simulink model "multiRobotExampleModel"  (R2019b)
settings: Solver=FixedStepAuto  StartTime=0.0  StopTime=inf  FixedStep=0.1  RelTol=1e-3
PreLoadFcn:
  | exampleMultiRobotHelperInit
InitFcn:
  | set_param('multiRobotExampleModel', 'ForceConsistencyChecking', 'off');
undefined symbols (not defined in the file): chargingStations, loadingStation, logicalMap, numRobots, packages, RobotState, unloadingStations
libraries: robotmobilelib x5
settings Model: Creator=The MathWorks, Inc.  LastModifiedBy=Helsi

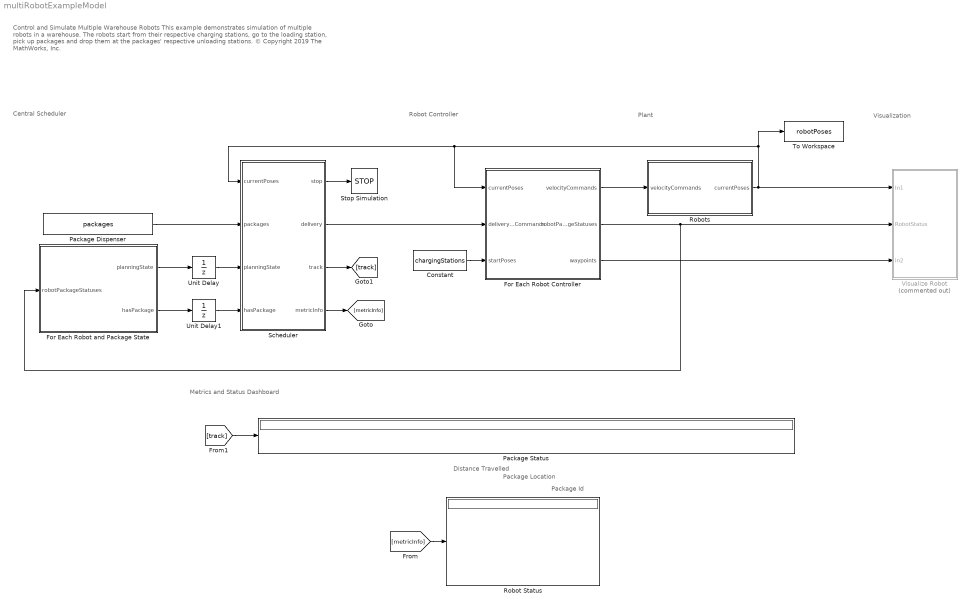
== system multiRobotExampleModel ==
  note: Visualization
  note: Plant
  note: Robot Controller
  note: Central Scheduler
  note: Metrics and Status Dashboard
  note: Package
      | Location
  note: Package Id
  note: Distance
      | Travelled
  note: Control and Simulate Multiple Warehouse Robots
      | This example demonstrates simulation of multiple robots in a warehouse. The robots start from their respective charging stations, go to the loading station, pick up packages and drop them at the packages' respective unloading stations.
      |
      | © Copyright 2019 The MathWorks, Inc.
  Constant : Constant  Value=chargingStations
  For Each Robot Controller : Subsystem  TreatAsAtomicUnit=on
  For Each Robot and Package State : Subsystem  TreatAsAtomicUnit=on
  Package Dispenser : Constant  Value=packages
  "Package Status " : Display
  Robot Status : Display
  Robots : Subsystem
  Scheduler : Stateflow chart  Priority=1  BlockKeywords=__PRM__SERIALIZED__DATA__:Stateflow Chart,Stateflow Diagram  TreatAsAtomicUnit=on
  Stop Simulation : Stop
  To Workspace : ToWorkspace  VariableName=robotPoses  SampleTime=-1
  Unit Delay : UnitDelay  InitialCondition=repmat(RobotState.AtDock, [1, numRobots])  SampleTime=-1  HasFrameUpgradeWarning=on
  Unit Delay1 : UnitDelay  InitialCondition=repmat(0, [1, numRobots])  SampleTime=-1  HasFrameUpgradeWarning=on
  Visualize Robot : Subsystem  Commented=on  mask{MeshSelectionIdx=Ground vehicle, PresetViews=Entire Map, ShowViz=on, ShowPaths=on, MapXMin=0, MapXMax=[], MapYMin=0, MapYMax=[], XLimits=[0 60], YLimits=[0 60], LocalXLimits=[-10 10], LocalYLimits=[-10 10], StartLocations=chargingStations, DockLocations=loadingStation, ShelfLocations=unloadingStations, VisualizationSampleRate=10}
      mask prompts: MeshSelectionIdx "Robot mesh"; PresetViews "Preset Views"; ShowViz "Update visualization:"; ShowPaths "Show planned paths:"; MapXMin "Map xmin:"; MapXMax "Map xmax:"; MapYMin "Map ymin:"; MapYMax "Map ymax:"; XLimits "Map x-limits:"; YLimits "Map y-limits:"; LocalXLimits "Local view x-limits"; LocalYLimits "Local view y-limits"; StartLocations "Start locations:"; DockLocations "Dock locations:"; ShelfLocations "Shelf locations:"; VisualizationSampleRate "Sample time:"
      mask init:
      | % Create the list of key locations
      | startLocationMatrix = evalin('base', get_param(gcb, 'StartLocations'));
      | shelfLocationMatrix = evalin('base', get_param(gcb, 'ShelfLocations'));
      | dockLocationMatrix = evalin('base', get_param(gcb, 'DockLocations'));
      | 
      | % Create popup list from matrices
      | dockLocationNameCell = cell(size(dockLocationMatrix,1),1);
      | shelfLocationNameCell = cell(size(shelfLocationMatrix,1),1);
      | startLocationNameCell = cell(size(startLocationMatrix,1),1);
      | for i = 1:size(startLocationMatrix,1)
      |     startLocationNameCell{i} = ['Start Location ' num2str(i)];
      | end
      | for j = 1:size(shelfLocationMatrix,1)
      |     shelfLocationNameCell{j} = ['Shelf Location ' num2str(j)];
      | end
      | for k = 1:size(dockLocationMatrix,1)
      |     dockLocationNameCell{k} = ['Dock Location ' num2str(k)];
      | end
      | 
      | % Update the parameter list
      | m = Simulink.Mask.get(gcb);
      | viewPopupParam = m.getParameter('PresetViews');
      | viewPopupParam.TypeOptions = [...
      |     {'Entire Map'}; ...
      |     dockLocationNameCell; ...
      |     shelfLocationNameCell; ...
      |     startLocationNameCell ... 
      |     ];
      mask TypeOptions MeshSelectionIdx: Ground vehicle | Forklift
      mask TypeOptions PresetViews: Entire Map | Dock Location 1 | Shelf Location 1 | Shelf Location 2 | Shelf Location 3 | Start Location 1 | Start Location 2 | Start Location 3 | Start Location 4 | Start Location 5
      mask Callback PresetViews:
      | % Get key numeric data
      | startLocationMatrix = evalin('base', get_param(gcb, 'StartLocations'));
      | dockLocationMatrix = evalin('base', get_param(gcb, 'DockLocations'));
      | shelfLocationMatrix = evalin('base', get_param(gcb, 'ShelfLocations'));
      | mapXLim = evalin('base', get_param(gcb, 'XLimits'));
      | mapYLim = evalin('base', get_param(gcb, 'YLimits'));
      | viewXLim = evalin('base', get_param(gcb, 'LocalXLimits'));
      | viewYLim = evalin('base', get_param(gcb, 'LocalYLimits'));
      | 
      | % Get selected value
      | viewSelection = get_param(gcb, 'PresetViews');
      | 
      | % Take action based on view
      | if strcmp(viewSelection, 'Custom')
      |     % Do nothing
      | else
      |     if strcmp(viewSelection(1:5), 'Start')
      |         % Start location
      |         startIndex = str2double(viewSelection(16:end));
      |         localPts = startLocationMatrix(startIndex, :);
      |         viewLimits = [localPts(1)+viewXLim(1) localPts(1)+viewXLim(2) ...
      |             localPts(2)+viewYLim(1) localPts(2)+viewYLim(2)];
      | 
      |     elseif strcmp(viewSelection(1:5), 'Dock ')
      |         % Dock (Loading) location
      |         dockIndex = str2double(viewSelection(15:end));
      |         localPts = dockLocationMatrix(dockIndex, :);
      |         viewLimits = [localPts(1)+viewXLim(1) localPts(1)+viewXLim(2) ...
      |             localPts(2)+viewYLim(1) localPts(2)+viewYLim(2)];
      | 
      |     elseif strcmp(viewSelection(1:5), 'Shelf')
      |         % Shelf (Unloading) location
      |         shelfIndex = str2double(viewSelection(16:end));
      |         localPts = shelfLocationMatrix(shelfIndex, :);
      |         viewLimits = [localPts(1)+viewXLim(1) localPts(1)+viewXLim(2) ...
      |             localPts(2)+viewYLim(1) localPts(2)+viewYLim(2)];
      | 
      |     else
      |         % Show the whole map
      |         viewLimits = [mapXLim(1) mapXLim(2) mapYLim(1) mapYLim(2)];
      |     end
      | 
      |     % Set the map parameters
      |     set_param(gcb, 'MapXMin', num2str(viewLimits(1)));
      |     set_param(gcb, 'MapXMax', num2str(viewLimits(2)));
      |     set_param(gcb, 'MapYMin', num2str(viewLimits(3)));
      |     set_param(gcb, 'MapYMax', num2str(viewLimits(4)));
      | end
      mask Callback MapXMin:
      | currentMax = str2num(get_param(gcb, 'MapXMax'));
      | newMin = str2num(get_param(gcb, 'MapXMin'));
      | if newMin > currentMax
      |     set_param(gcb, 'MapXMax', num2str(newMin+1));
      | end
      mask Callback MapXMax:
      | currentMin = str2num(get_param(gcb, 'MapXMin'));
      | newMax = str2num(get_param(gcb, 'MapXMax'));
      | if newMax < currentMin
      |     set_param(gcb, 'MapXMin', num2str(newMax-1));
      | end
      mask Callback MapYMin:
      | currentMax = str2num(get_param(gcb, 'MapYMax'));
      | newMin = str2num(get_param(gcb, 'MapYMin'));
      | if newMin > currentMax
      |     set_param(gcb, 'MapYMax', num2str(newMin+1));
      | end
      mask Callback MapYMax:
      | currentMin = str2num(get_param(gcb, 'MapYMin'));
      | newMax = str2num(get_param(gcb, 'MapYMax'));
      | if newMax < currentMin
      |     set_param(gcb, 'MapYMin', num2str(newMax-1));
      | end
      mask DialogControl DescGroupVar Prompt: Visualization example helper
      mask DialogControl DescTextVar Prompt: This subsystem plots the robots and environement and allows users to change the views.
      mask DialogControl ViewLimits Prompt: View limits
      mask DialogControl ViewConfigurationGroup Prompt: View configuration:
      mask DialogControl ViewParamSourcesGroup Prompt: View parameter sources
      mask Display: disp('Visualization Helper')
  wires:
  For Each Robot and Package State/2(hasPackage) -> Unit Delay1/1
  For Each Robot and Package State/1(planningState) -> Unit Delay/1
  Package Dispenser/1 -> Scheduler/2(packages)
  Scheduler/2(delivery) -> For Each Robot Controller/2(deliveryCommands)
  Scheduler/1(stop) -> Stop Simulation/1
  Unit Delay1/1 -> Scheduler/4(hasPackage)
  [track] -> "Package Status "/1
  For Each Robot Controller/2(robotPackageStatuses) -> For Each Robot and Package State/1(robotPackageStatuses), Visualize Robot/2(RobotStatus)
  Scheduler/4(metricInfo) -> [metricInfo]
  For Each Robot Controller/3(waypoints) -> Visualize Robot/3(In2)
  [metricInfo] -> Robot Status/1
  For Each Robot Controller/1(velocityCommands) -> Robots/1(velocityCommands)
  Scheduler/3(track) -> [track]
  Unit Delay/1 -> Scheduler/3(planningState)
  Constant/1 -> For Each Robot Controller/3(startPoses)
  Robots/1(currentPoses) -> Visualize Robot/1(In1), To Workspace/1, For Each Robot Controller/1(currentPoses), Scheduler/1(currentPoses)

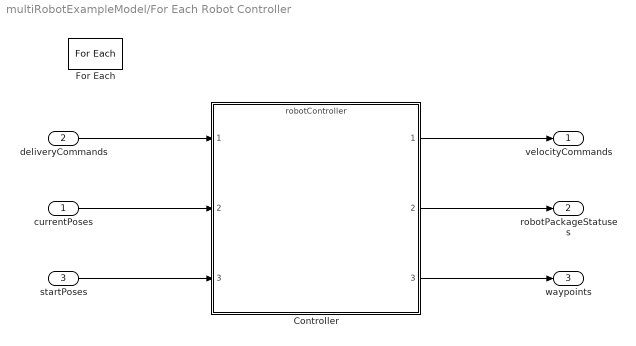
== system multiRobotExampleModel/For Each Robot Controller ==
  currentPoses : Inport  Partition=on  PartitionDimension=2  PartitionWidth=1  PartitionOffset=0
  deliveryCommands : Inport  Port=2  Partition=on  PartitionDimension=1  PartitionWidth=1  PartitionOffset=0
  startPoses : Inport  Port=3  Partition=on  PartitionDimension=1  PartitionWidth=1  PartitionOffset=0
  Controller : ModelReference  ModelNameDialog=robotController.slx  ModelReferenceVersion=1.116
  For Each : ForEach  DisableCoverage=on
  velocityCommands : Outport  ConcatenationDimension=2
  robotPackageStatuses : Outport  Port=2  ConcatenationDimension=1
  waypoints : Outport  Port=3  ConcatenationDimension=3
  wires:
  deliveryCommands/1 -> Controller/1
  currentPoses/1 -> Controller/2
  startPoses/1 -> Controller/3
  Controller/1 -> velocityCommands/1
  Controller/2 -> robotPackageStatuses/1
  Controller/3 -> waypoints/1

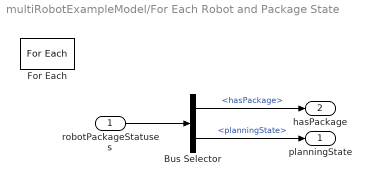
== system multiRobotExampleModel/For Each Robot and Package State ==
  robotPackageStatuses : Inport  Partition=on  PartitionDimension=1  PartitionWidth=1  PartitionOffset=0
  Bus Selector : BusSelector  OutputSignals=hasPackage,planningState
  For Each : ForEach  DisableCoverage=on
  planningState : Outport  ConcatenationDimension=1
  hasPackage : Outport  Port=2  ConcatenationDimension=1
  wires:
  robotPackageStatuses/1 -> Bus Selector/1
  Bus Selector/1 -> hasPackage/1  "<hasPackage>"
  Bus Selector/2 -> planningState/1  "<planningState>"

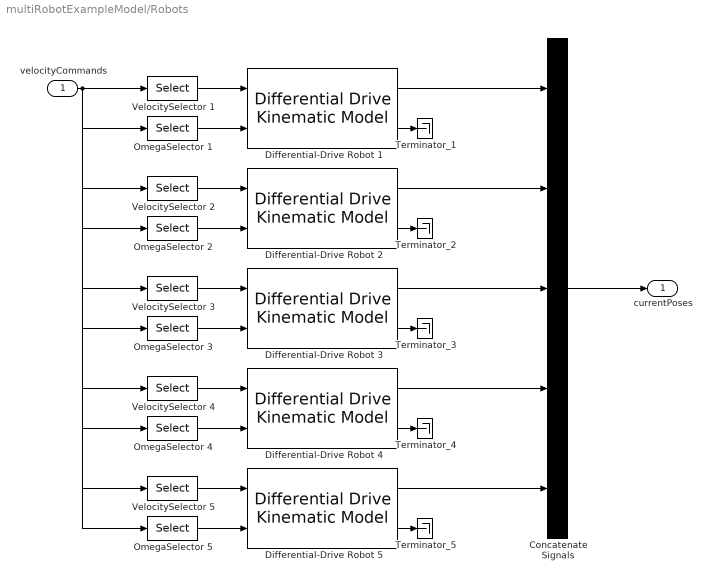
== system multiRobotExampleModel/Robots ==
  velocityCommands : Inport
  Concatenate Signals : Concatenate  NumInputs=5  Mode=Multidimensional array  ConcatenateDimension=2
  Differential-Drive Robot 1 : robotmobilelib/Differential Drive Kinematic Model  VehicleInputs=Vehicle Speed & Heading Angular Velocity  WheelRadius=0.1  WheelSpeedRange=[-inf inf]  TrackWidth=0.2  InitialState=[chargingStations(1, :), 0]'  SimulateUsing=Interpreted execution
      settings: SourceProductName=Robotics System Toolbox  SourceProductBaseCode=RO
  Differential-Drive Robot 2 : robotmobilelib/Differential Drive Kinematic Model  VehicleInputs=Vehicle Speed & Heading Angular Velocity  WheelRadius=0.1  WheelSpeedRange=[-inf inf]  TrackWidth=0.2  InitialState=[chargingStations(2, :), 0]'  SimulateUsing=Interpreted execution
      settings: SourceProductName=Robotics System Toolbox  SourceProductBaseCode=RO
  Differential-Drive Robot 3 : robotmobilelib/Differential Drive Kinematic Model  VehicleInputs=Vehicle Speed & Heading Angular Velocity  WheelRadius=0.1  WheelSpeedRange=[-inf inf]  TrackWidth=0.2  InitialState=[chargingStations(3, :), 0]'  SimulateUsing=Interpreted execution
      settings: SourceProductName=Robotics System Toolbox  SourceProductBaseCode=RO
  Differential-Drive Robot 4 : robotmobilelib/Differential Drive Kinematic Model  VehicleInputs=Vehicle Speed & Heading Angular Velocity  WheelRadius=0.1  WheelSpeedRange=[-inf inf]  TrackWidth=0.2  InitialState=[chargingStations(4, :), 0]'  SimulateUsing=Interpreted execution
      settings: SourceProductName=Robotics System Toolbox  SourceProductBaseCode=RO
  Differential-Drive Robot 5 : robotmobilelib/Differential Drive Kinematic Model  VehicleInputs=Vehicle Speed & Heading Angular Velocity  WheelRadius=0.1  WheelSpeedRange=[-inf inf]  TrackWidth=0.2  InitialState=[chargingStations(5, :), 0]'  SimulateUsing=Interpreted execution
      settings: SourceProductName=Robotics System Toolbox  SourceProductBaseCode=RO
  OmegaSelector 1 : Selector  NumberOfDimensions=2  InputPortWidth=3  IndexOptions=Index vector (dialog),Index vector (dialog)  Indices=2,1  OutputSizes=1
  OmegaSelector 2 : Selector  NumberOfDimensions=2  InputPortWidth=3  IndexOptions=Index vector (dialog),Index vector (dialog)  Indices=2,2  OutputSizes=1
  OmegaSelector 3 : Selector  NumberOfDimensions=2  InputPortWidth=3  IndexOptions=Index vector (dialog),Index vector (dialog)  Indices=2,3  OutputSizes=1
  OmegaSelector 4 : Selector  NumberOfDimensions=2  InputPortWidth=3  IndexOptions=Index vector (dialog),Index vector (dialog)  Indices=2,4  OutputSizes=1
  OmegaSelector 5 : Selector  NumberOfDimensions=2  InputPortWidth=3  IndexOptions=Index vector (dialog),Index vector (dialog)  Indices=2,5  OutputSizes=1
  Terminator_{1..5} (5 alike) : Terminator
  VelocitySelector 1 : Selector  NumberOfDimensions=2  InputPortWidth=3  IndexOptions=Index vector (dialog),Index vector (dialog)  Indices=1,1  OutputSizes=1
  VelocitySelector 2 : Selector  NumberOfDimensions=2  InputPortWidth=3  IndexOptions=Index vector (dialog),Index vector (dialog)  Indices=1,2  OutputSizes=1
  VelocitySelector 3 : Selector  NumberOfDimensions=2  InputPortWidth=3  IndexOptions=Index vector (dialog),Index vector (dialog)  Indices=1,3  OutputSizes=1
  VelocitySelector 4 : Selector  NumberOfDimensions=2  InputPortWidth=3  IndexOptions=Index vector (dialog),Index vector (dialog)  Indices=1,4  OutputSizes=1
  VelocitySelector 5 : Selector  NumberOfDimensions=2  InputPortWidth=3  IndexOptions=Index vector (dialog),Index vector (dialog)  Indices=1,5  OutputSizes=1
  currentPoses : Outport
  wires:
  Concatenate Signals/1 -> currentPoses/1
  velocityCommands/1 -> VelocitySelector 1/1, OmegaSelector 1/1, VelocitySelector 2/1, OmegaSelector 2/1, VelocitySelector 3/1, OmegaSelector 3/1, VelocitySelector 4/1, OmegaSelector 4/1, VelocitySelector 5/1, OmegaSelector 5/1
  VelocitySelector 1/1 -> Differential-Drive Robot 1/1
  OmegaSelector 1/1 -> Differential-Drive Robot 1/2
  Differential-Drive Robot 1/1 -> Concatenate Signals/1
  VelocitySelector 2/1 -> Differential-Drive Robot 2/1
  OmegaSelector 2/1 -> Differential-Drive Robot 2/2
  Differential-Drive Robot 2/1 -> Concatenate Signals/2
  VelocitySelector 3/1 -> Differential-Drive Robot 3/1
  OmegaSelector 3/1 -> Differential-Drive Robot 3/2
  Differential-Drive Robot 3/1 -> Concatenate Signals/3
  VelocitySelector 4/1 -> Differential-Drive Robot 4/1
  OmegaSelector 4/1 -> Differential-Drive Robot 4/2
  Differential-Drive Robot 4/1 -> Concatenate Signals/4
  VelocitySelector 5/1 -> Differential-Drive Robot 5/1
  OmegaSelector 5/1 -> Differential-Drive Robot 5/2
  Differential-Drive Robot 5/1 -> Concatenate Signals/5
  Differential-Drive Robot 1/2 -> Terminator_1/1
  Differential-Drive Robot 2/2 -> Terminator_2/1
  Differential-Drive Robot 3/2 -> Terminator_3/1
  Differential-Drive Robot 4/2 -> Terminator_4/1
  Differential-Drive Robot 5/2 -> Terminator_5/1

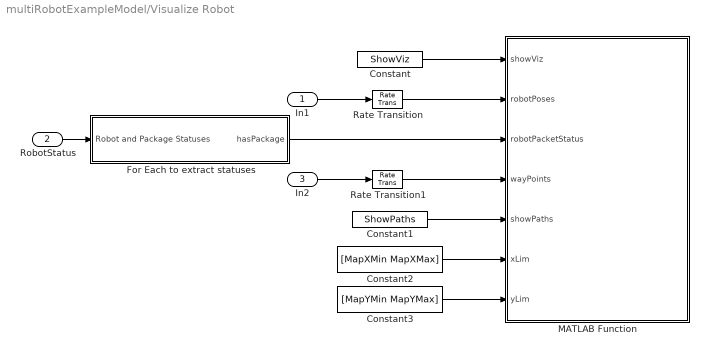
== system multiRobotExampleModel/Visualize Robot ==
  In1 : Inport
  RobotStatus : Inport  Port=2
  In2 : Inport  Port=3
  Constant : Constant  Value=ShowViz
  Constant1 : Constant  Value=ShowPaths
  Constant2 : Constant  Value=[MapXMin MapXMax]
  Constant3 : Constant  Value=[MapYMin MapYMax]
  For Each to extract statuses : Subsystem  TreatAsAtomicUnit=on
  MATLAB Function : MATLAB Function  TreatAsAtomicUnit=on
  Rate Transition : RateTransition
  Rate Transition1 : RateTransition
  wires:
  In2/1 -> Rate Transition1/1
  In1/1 -> Rate Transition/1
  Rate Transition/1 -> MATLAB Function/2(robotPoses)
  Rate Transition1/1 -> MATLAB Function/4(wayPoints)
  Constant/1 -> MATLAB Function/1(showViz)
  Constant1/1 -> MATLAB Function/5(showPaths)
  Constant2/1 -> MATLAB Function/6(xLim)
  Constant3/1 -> MATLAB Function/7(yLim)
  RobotStatus/1 -> For Each to extract statuses/1(Robot and Package Statuses)
  For Each to extract statuses/1(hasPackage) -> MATLAB Function/3(robotPacketStatus)

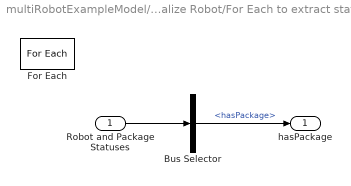
== system multiRobotExampleModel/Visualize Robot/For Each to extract statuses ==
  Robot and Package Statuses : Inport  Partition=on  PartitionDimension=1  PartitionWidth=1  PartitionOffset=0
  Bus Selector : BusSelector  OutputSignals=hasPackage
  For Each : ForEach  DisableCoverage=on
  hasPackage : Outport  ConcatenationDimension=1
  wires:
  Robot and Package Statuses/1 -> Bus Selector/1
  Bus Selector/1 -> hasPackage/1  "<hasPackage>"

== matlab function multiRobotExampleModel/Visualize Robot/MATLAB Function ==
  settings: updateMethod=DISCRETE  sampleTime=VisualizationSampleRate
  data: showViz input; robotPoses input; robotPacketStatus input; wayPoints input; logicalMap parameter; ShelfLocations parameter; DockLocations parameter; showPaths input; xLim input; yLim input; MeshSelectionIdx parameter
function simulationVisualization(showViz, robotPoses, robotPacketStatus, wayPoints, logicalMap, ShelfLocations, DockLocations, showPaths, xLim, yLim, MeshSelectionIdx)
%#codegen

%% Setup

coder.extrinsic('exampleHelperVisualizeWarehouseRobots');
persistent f ax

if isempty(f) && showViz
    f = figure('units','normalized','outerposition',[0 0 0.75 0.75]);
    ax = axes('Parent', f);
    title('Mobile Robot Motion');
    set(f, 'Visible', 'on');
end

% Robot mesh options are cells of the unloaded and loaded robot mesh and
% the translation between the visualized origin and the desired origin
meshOptions = {...
    {'groundvehicle.stl', [.314 0 .155], 'groundvehiclewithload.stl', [.312 0 .156]}, ...
    {'forklift.stl', [.3569 0 .297], 'forkliftwithload.stl', [.3813 0 .2893]}, ...
    };
    

if showViz
    exampleHelperVisualizeWarehouseRobots(robotPoses, robotPacketStatus, wayPoints, logicalMap, ShelfLocations, DockLocations, showPaths, xLim, yLim, meshOptions{MeshSelectionIdx});
end

end

== stateflow chart multiRobotExampleModel/Scheduler ==
  settings: sampleTime=0.1
  state Assign
    entry:
    stop = 0;
    entry, during:
    activeRobots = avoidCollision(currentPoses, collisionThresh);
    Assign -> (junction 258) [order 1] : [currentPackage <= length(packages)]{robot = 1;}
    (junction 258) -> (junction 257) [order 1] : [robot <= numRobots]{delivery(robot).active = activeRobots(robot);}
    (junction 257) -> (junction 391) [order 1] : [planningState(robot) == RobotState.AtLoadingStn && ...
        | ~hasPackage(robot)&&...
        | currentPackage <= length(packages)]
        | {
        | delivery(robot).package= packages(currentPackage);
        | delivery(robot).packageId = currentPackage;
        | currentPackage = currentPackage + 1;
        | delivery(robot).givenPackage = 1;
        | }
    (junction 258) -> (junction 398) [order 2] : {packageTrack;
        | robotTrack;}
    (junction 393) -> (junction 258)
    (junction 257) -> (junction 259) [order 2] : {delivery(robot).givenPackage = 0;}
    (junction 391) -> (junction 332)
    (junction 259) -> (junction 393) : {robot = robot + 1;}
    (junction 332) -> (junction 259)
  state LastPackage
    entry, during:
    activeRobots = avoidCollision(currentPoses, collisionThresh);
    LastPackage -> (junction 344) [order 1] : {robot = 1;}
    (junction 344) -> (junction 343) [order 1] : [robot <= numRobots]{delivery(robot).active = activeRobots(robot);}
    (junction 344) -> (junction 426) [order 2] : {packageTrack;
        | robotTrack;}
    (junction 346) -> (junction 344)
    (junction 343) -> (junction 345) : {delivery(robot).givenPackage = 0;
        | }
    (junction 345) -> (junction 346) : {robot = robot + 1;}
  state Stop
    stop = 1;
  (default) -> Assign
  Assign -> LastPackage [order 1] : [currentPackage > length(packages)]
      | {packageTrack;
      | robotTrack;}
  Stop -> (junction 351)
  LastPackage -> Stop [order 1] : [~any(hasPackage)]{
      | robotTrack;
      | packageTrack;}
  data: robotActive function_output size=[1, numRobots]; robotPoses function_input double size=[3, numRobots]; thresh function_input size=[1. 1]; currentPoses input; packages input; planningState input; robot local =1; stop output; currentPackage local =1; hasPackage input; numRobots local =size(chargingStations, 1); delivery output Bus: RobotDeliverCommand size=numRobots; activeRobots local size=[1, numRobots] =ones(1, numRobots); collisionThresh parameter; track output Enum: PackageState size=[1, length(packets)] =repmat(PackageState.Unassigned, 1, length(packages)); prevPose local =chargingStations'; metricInfo output =zeros(numRobots, 3); distance local =zeros(numRobots, 1)
  function robotActive = avoidCollision(robotPoses,thresh):
    | function robotActive = avoidCollision(robotPoses,thresh)
    | nRobots = size(robotPoses, 2);
    | robotActive = ones(1, nRobots);
    | poseIdx = 1:2;
    | 
    | % calculate robot pairwise distances
    | poses = robotPoses(poseIdx, :)';
    | robotPairwiseDistances = zeros(nRobots, nRobots);
    | robotPairwiseDistances = exampleHelperRobotPairwiseDistances(poses, poses);
    | 
    | % check if robots are too close
    | robotCollisions = robotPairwiseDistances < thresh;
    | for i = 1:nRobots
    |     robotActive(i) = ~any(find(robotCollisions(i, :)) < i);
    | end
    | end
  function packageTrack:
    | function packageTrack
    | numPackets = length(packages);
    | for r = 1 : numRobots
    |     packageId = delivery(r).packageId;
    |     if(packageId > 0 && track(packageId) ~= PackageState.Delivered)
    |         track(packageId) = PackageState.InProgress;
    |     end
    |     if(packageId > 0)
    |         if(~hasPackage(r) && planningState(r) == RobotState.AtUnloadingStn)
    |             track(packageId) = PackageState.Delivered;
    |         end
    |     end
    | end
  function robotTrack:
    | function robotTrack
    | % calculate distance
    | displacement = (prevPose - currentPoses(1:2, :));
    | d = sqrt(diag(displacement' * displacement));
    | distance = distance + d;
    | prevPose = currentPoses(1:2, :);
    | d = distance;
    | metricInfo(:, 1) = distance(:);
    | 
    | robotPackages = zeros(1, numRobots);
    | robotPackageId = zeros(1, numRobots);
    | packetIds = zeros(1, numRobots);
    | for r = 1:numRobots
    |     robotPackages(r) = delivery(r).package;
    |     robotPackageId(r) = delivery(r).packageId;
    | end
    | metricInfo(:, 2) = robotPackages(:);
    | metricInfo(:, 3) = robotPackageId(:);
    | end
